simulink model "SimulazioneCaso2"  (R2019b)
settings: Solver=VariableStepAuto  StartTime=0.0  StopTime=100  RelTol=1e-3
libraries: simulink x2
settings Model: Creator=sugam  LastModifiedBy=sugam

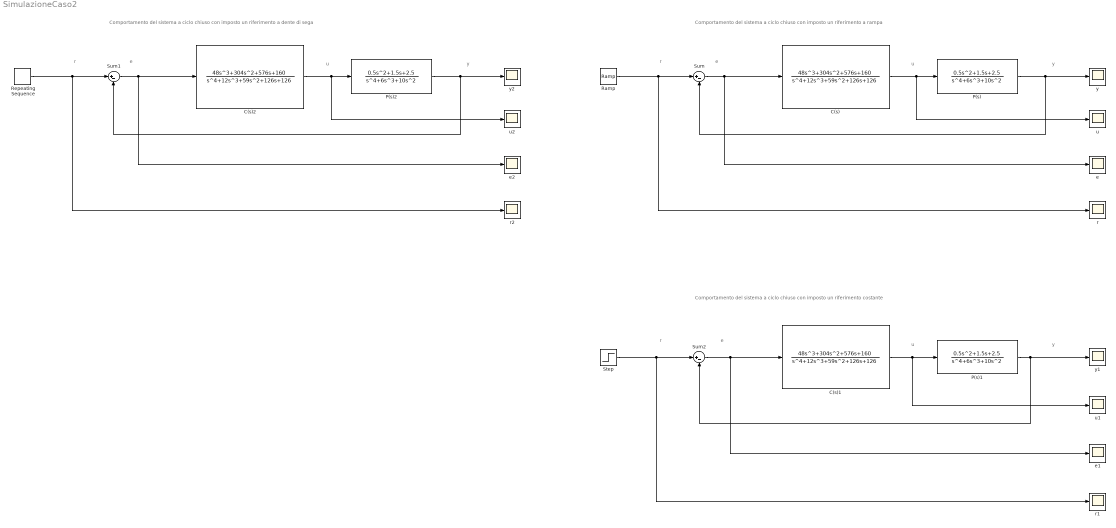
== system SimulazioneCaso2 ==
  note: Comportamento del sistema a ciclo chiuso con imposto un riferimento a dente di sega
  note: y
  note: u
  note: r
  note: e
  note: e
  note: r
  note: y
  note: u
  note: r
  note: e
  note: u
  note: y
  note: Comportamento del sistema a ciclo chiuso con imposto un riferimento a rampa
  note: Comportamento del sistema a ciclo chiuso con imposto un riferimento costante
  C(s) : TransferFcn  Numerator=[0 48 304 576 160]  Denominator=[1 12 59 126 126]
  C(s)1 : TransferFcn  Numerator=[0 48 304 576 160]  Denominator=[1 12 59 126 126]
  C(s)2 : TransferFcn  Numerator=[0 48 304 576 160]  Denominator=[1 12 59 126 126]
  P(s) : TransferFcn  Numerator=[0.5 1.5 2.5]  Denominator=[1 6 10 0 0]
  P(s)1 : TransferFcn  Numerator=[0.5 1.5 2.5]  Denominator=[1 6 10 0 0]
  P(s)2 : TransferFcn  Numerator=[0.5 1.5 2.5]  Denominator=[1 6 10 0 0]
  Ramp : simulink/Sources/Ramp  slope=1  start=0  InitialOutput=0
  Repeating Sequence : simulink/Sources/Repeating Sequence  rep_seq_t=[0 5]  rep_seq_y=[0 10]
  Step : Step  After=10  SampleTime=0
  Sum : Sum  Inputs=|+-
  Sum1 : Sum  Inputs=|+-
  Sum2 : Sum  Inputs=|+-
  e : Scope
  e1 : Scope
  e2 : Scope
  r : Scope
  r1 : Scope
  r2 : Scope
  u : Scope
  u1 : Scope
  u2 : Scope
  y : Scope
  y1 : Scope
  y2 : Scope
  wires:
  P(s)/1 -> Sum/2, y/1
  Sum/1 -> e/1, C(s)/1
  C(s)/1 -> u/1, P(s)/1
  Step/1 -> r1/1, Sum2/1
  Ramp/1 -> r/1, Sum/1
  Sum2/1 -> e1/1, C(s)1/1
  C(s)1/1 -> u1/1, P(s)1/1
  P(s)1/1 -> y1/1, Sum2/2
  Repeating Sequence/1 -> r2/1, Sum1/1
  Sum1/1 -> e2/1, C(s)2/1
  P(s)2/1 -> Sum1/2, y2/1
  C(s)2/1 -> u2/1, P(s)2/1
